simulink model "IntecoVirtualDrl"  (R2020b)
settings: Solver=ode5  StartTime=0.0  StopTime=inf  FixedStep=0.01  RelTol=1e-3  AbsTol=1e-6
undefined symbols (not defined in the file): Standard_Devices, UDP_Protocol
libraries: sldrtlib x3, simulink x1
settings Model: SimulationMode=external  ExtModeTrigDuration=18000  ExtModeTrigLevel=0.400000  Creator=jims  LastModifiedBy=Mark
settings SolverCC: AutoScaleAbsTol=off
settings DataIOCC: ExternalInput=[]  InitialState=[]  MaxDataPoints=5000  SaveFormat=Array  SignalLoggingSaveFormat=ModelDataLogs  SaveOutput=off  SaveTime=off  ReturnWorkspaceOutputs=off
settings OptimizationCC: BooleanDataType=off  ExpressionDepthLimit=2147483647  LifeSpan=inf
settings DebuggingCC: SaveWithParameterizedLinksMsg=none  UnderspecifiedInitializationDetection=Classic  MergeDetectMultiDrivingBlocksExec=none  SignalResolutionControl=TryResolveAllWithWarning  MultiTaskDSMMsg=warning  MultiTaskCondExecSysMsg=none  IntegerOverflowMsg=none  FcnCallInpInsideContextMsg=warning  StateNameClashWarn=warning  SFUnexpectedBacktrackingDiag=warning  SFNoUnconditionalDefaultTransitionDiag=warning  SFExecutionAtInitializationDiag=none  IntegerSaturationMsg=none  ArithmeticOperatorsInVariantConditions=warning
settings HardwareCC: TargetBitPerLong=64  TargetBitPerPointer=64  TargetIntDivRoundTo=Zero  TargetEndianess=LittleEndian  TargetWordSize=64  TargetHWDeviceType=Intel->x86-64
settings ModelReferenceCC: PropagateSignalLabelsOutOfModel=off
settings SFSimCC: SimUseLocalCustomCode=off  CustomCodeUndefinedFunction=UseInterfaceOnly
settings RTWCC: Description=Simulink Desktop Real-Time  SystemTargetFile=sldrt.tlc  TemplateMakefile=sldrt.tmf  RTWUseLocalCustomCode=off  RTWCompilerOptimization=on
settings CodeAppCC: MaxIdLength=95  StateflowObjectComments=on
settings SimulinkDesktopRealTimeCC: TargetPreCompLibLocation=C:\Program Files\MATLAB\R2020b\toolbox\sldrt\lib\win64  TargetLangStandard=C89/C90 (ANSI)  SupportVariableSizeSignals=off
settings ConfigComp: CovMetricSettings=dw  CovSaveCumulativeToWorkspaceVar=on  CovSaveSingleToWorkspaceVar=on  CovExternalEMLEnable=off

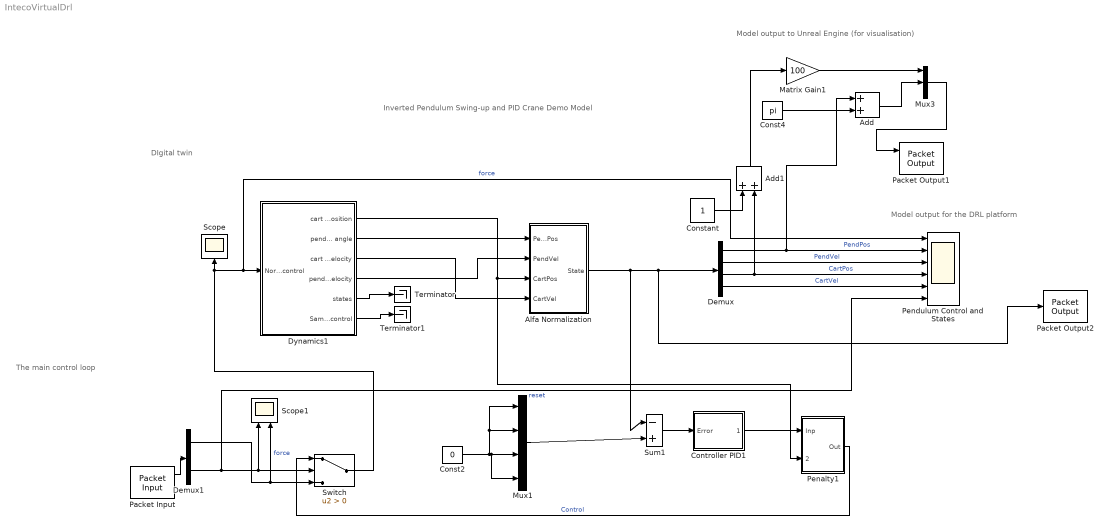
== system IntecoVirtualDrl ==
  note: Model output for the DRL platform
  note: Model output to Unreal Engine (for visualisation)
  note: DIgital twin
  note: The main control loop
  note: Inverted Pendulum
      | Swing-up and PID Crane Demo Model
  Add : Sum
  Add1 : Sum
  Alfa Normalization : Subsystem  mask(Choose mode:){}
  Const2 : Constant  Value=0
  Const4 : Constant  Value=pi
  Constant : Constant
  Controller PID1 : Subsystem  mask{Cart_PID=[ -0.8 0 -0.05 ], Pend_PID=[ -1 0 -0.0 ], Umax=0.5, zone=1.3, Friction=0.05, T0=0.01}
      mask prompts: Cart_PID "Cart PID parameters [Kp, Ki, Kd]:"; Pend_PID "Pendulum PID parameters [Kp, Ki, Kd]:"; Umax "Maximum control value:"; zone "Stabilisation zone [rad]:"; Friction "Friction compensation:"; T0 "Sample time:"
  Demux : Demux
      settings: DisplayOption=none
  Demux1 : Demux  Outputs=2
      settings: DisplayOption=none
  Dynamics1 : Subsystem  mask(Dynamics){x_ini=[0, 3.132388768862475, 0.002930656000000, 0.003140672265117062], m=[0.572066, 0.119648], fr=[0.000276, 1.199442, 0.502926], P4=[0.019631, 0.003861, 9.826466], Up=[6.338787, 0.227417], DZ=[0.099952, 1.495618]}
      mask prompts: x_ini "Initial state vector [x1(0)  x2(0)  x3(0)  x4(0)]"; m "mass of cart (mc)  mass of pendulum (mp)"; fr "friction :  fp  FS  FC"; P4 "Distance (l), Total Inertia moment (J), gravity (g)"; Up "control : magnitude (M)    DZu"; DZ "minimal velocities : cart (DZcv)  pendulum (DZcp)"
      mask help:
      | Pendulum-Cart Dynamics
      |
      | Copyright INTECO 1997
      mask init:
      | DZcv=DZ(1);DZcp=DZ(2);DZu=Up(2);l=P4(1);J=P4(2);g=P4(3);M=Up(1);mc=m(1);mp=m(2);fp=fr(1);FS=fr(2);FC=fr(3);mi=l*(mc+mp);a=l*l+J/(mc+mp);
      mask Display: plot(0,0,100,100,[40,48,48,40,40],[60,60,49,49,60],[37,44],[9,54],[100,8,4,1,0,100,100,0,40,100,100,0,0,40],[44,44,44,44,45,46,45,44,45,45,43,43,46,46],[100,48],[55,55],[0,40],[55,55])
  Matrix Gain1 : Gain  Gain=100  SaturateOnIntegerOverflow=on  OutDataTypeStr=Inherit: Same as input  ParamDataTypeStr=Inherit: Same as input
  Mux1 : Mux
  Mux3 : Mux  Inputs=3
  Packet Input : sldrtlib/Packet Input  SampleTime=0.03  MaxMissedTicks=10  ShowMissedTicks=off  YieldWhenWaiting=off  DrvName=Standard_Devices/UDP_Protocol  DrvAddress=16384  DrvOptions=[0 16384 49 50 55 46 48 46 48 46 49 0 0 0 0 0 0 0 0 0 0 0 0 0 0 0 0 0 0 0 0 0 0 0 0 0 0 0 0 0 0 0 0 0 0 0 0 0 0 0 0 0 0 0 0 0 0 0 0 0 0 0 0 0 0 0 0 0 0 0 0 0 0 0 0 0 0 0 0 0 0 0 0 0 0 0 0 0 0 0 0 0 0 0 0 0 0 0 0 0 0 0 0 0 0 0 0 0 0 0 0 0 0 0 0 0 0 0 0 0 0 0 0 0 0 0 0 0 0 0 0 0 0 0 0 0 0 0 0 0 0 0 0 0 0 0 0 0 0 0 0 0 0 0 0 0 0 0 0 0 0 0 0 0 0 0 0 0 0 0 0 0 0 0 0 0 0 0 0 0 0 0 0 0 0 0 0 0 0 0 0 0 0 0 0 0 0 0 0 0 0 0 0 0 0 0 0 0 0 0 0 0 0 0 0 0 0 0 0 0 0 0 0 0 0 0 0 0 0 0 0 0 0 0 0 0 0 0 0 0 0 0 0 0 0 0 0 0 0 0 0 0 0 0 0 0]  PacketSize=16  DataTypes='2*double'  ShowReady=on  ShowError=off  PacketID=1  ByteOrder=2  ShowTimestamp=off
      settings: AttributesFormatString=UDP Protocol [16384]
  Packet Output1 : sldrtlib/Packet Output  SampleTime=0.03  MaxMissedTicks=25  ShowMissedTicks=on  YieldWhenWaiting=off  DrvName=Standard_Devices/UDP_Protocol  DrvAddress=9999  DrvOptions=[0 8888 49 50 55 46 48 46 48 46 49 0 0 0 0 0 0 0 0 0 0 0 0 0 0 0 0 0 0 0 0 0 0 0 0 0 0 0 0 0 0 0 0 0 0 0 0 0 0 0 0 0 0 0 0 0 0 0 0 0 0 0 0 0 0 0 0 0 0 0 0 0 0 0 0 0 0 0 0 0 0 0 0 0 0 0 0 0 0 0 0 0 0 0 0 0 0 0 0 0 0 0 0 0 0 0 0 0 0 0 0 0 0 0 0 0 0 0 0 0 0 0 0 0 0 0 0 0 0 0 0 0 0 0 0 0 0 0 0 0 0 0 0 0 0 0 0 0 0 0 0 0 0 0 0 0 0 0 0 0 0 0 0 0 0 0 0 0 0 0 0 0 0 0 0 0 0 0 0 0 0 0 0 0 0 0 0 0 0 0 0 0 0 0 0 0 0 0 0 0 0 0 0 0 0 0 0 0 0 0 0 0 0 0 0 0 0 0 0 0 0 0 0 0 0 0 0 0 0 0 0 0 0 0 0 0 0 0 0 0 0 0 0 0 0 0 0 0 0 0 0 0 0 0 0 0]  PacketSize=83  DataTypes={'20*single', '3*uint8'}  ShowReady=off  ShowError=off  PacketID=1  ByteOrder=1  InitialValue=[]  FinalValue=[]
      settings: AttributesFormatString=UDP Protocol [9999]
  Packet Output2 : sldrtlib/Packet Output  SampleTime=0.03  MaxMissedTicks=25  ShowMissedTicks=on  YieldWhenWaiting=off  DrvName=Standard_Devices/UDP_Protocol  DrvAddress=16385  DrvOptions=[0 16385 49 50 55 46 48 46 48 46 49 0 0 0 0 0 0 0 0 0 0 0 0 0 0 0 0 0 0 0 0 0 0 0 0 0 0 0 0 0 0 0 0 0 0 0 0 0 0 0 0 0 0 0 0 0 0 0 0 0 0 0 0 0 0 0 0 0 0 0 0 0 0 0 0 0 0 0 0 0 0 0 0 0 0 0 0 0 0 0 0 0 0 0 0 0 0 0 0 0 0 0 0 0 0 0 0 0 0 0 0 0 0 0 0 0 0 0 0 0 0 0 0 0 0 0 0 0 0 0 0 0 0 0 0 0 0 0 0 0 0 0 0 0 0 0 0 0 0 0 0 0 0 0 0 0 0 0 0 0 0 0 0 0 0 0 0 0 0 0 0 0 0 0 0 0 0 0 0 0 0 0 0 0 0 0 0 0 0 0 0 0 0 0 0 0 0 0 0 0 0 0 0 0 0 0 0 0 0 0 0 0 0 0 0 0 0 0 0 0 0 0 0 0 0 0 0 0 0 0 0 0 0 0 0 0 0 0 0 0 0 0 0 0 0 0 0 0 0 0 0 0 0 0 0 0]  PacketSize=32  DataTypes='4*double'  ShowReady=off  ShowError=off  PacketID=1  ByteOrder=2  InitialValue=[]  FinalValue=[]
      settings: AttributesFormatString=UDP Protocol [16385]
  Penalty1 : Subsystem
  Pendulum Control and States : Scope  NumInputPorts=6
  Scope : Scope
  Scope1 : Scope  NumInputPorts=2
  Sum1 : Sum  Inputs=|-+  InputSameDT=on  SaturateOnIntegerOverflow=on  OutDataTypeStr=Inherit: Same as first input
  Switch : Switch  Criteria=u2 > Threshold
  Terminator : Terminator
  Terminator1 : Terminator
  wires:
  Demux/4 -> Pendulum Control and States/5  "CartVel"
  Demux/3 -> Pendulum Control and States/4, Add1/2  "CartPos"
  Demux/2 -> Pendulum Control and States/3  "PendVel"
  Demux/1 -> Add/1, Pendulum Control and States/2  "PendPos"
  Dynamics1/2(pendulum angle) -> Alfa Normalization/1(PendPos)
  Dynamics1/4(pendulum velocity) -> Alfa Normalization/2(PendVel)
  Dynamics1/1(cart position) -> Penalty1/2(CartPos), Alfa Normalization/3(CartPos)
  Dynamics1/3(cart velocity) -> Alfa Normalization/4(CartVel)
  Dynamics1/5(states) -> Terminator/1
  Dynamics1/6(Sampled control) -> Terminator1/1
  Mux3/1 -> Packet Output1/1
  Matrix Gain1/1 -> Mux3/1
  Const4/1 -> Add/2
  Add/1 -> Mux3/2
  Sum1/1 -> Controller PID1/1(Error)
  Packet Input/1 -> Demux1/1
  Demux1/2 -> Pendulum Control and States/6, Scope1/1, Switch/2  "reset"
  Demux1/1 -> Switch/3, Scope1/2  "force"
  Switch/1 -> Dynamics1/1(Normalized control), Pendulum Control and States/1, Scope/1  "force"
  Constant/1 -> Add1/1
  Add1/1 -> Matrix Gain1/1
  Const2/1 -> Mux1/1, Mux1/2, Mux1/4, Mux1/3
  Mux1/1 -> Sum1/2
  Controller PID1/1(Control) -> Penalty1/1(Inp)
  Alfa Normalization/1(State) -> Sum1/1, Packet Output2/1, Demux/1
  Penalty1/1(Out) -> Switch/1  "Control"

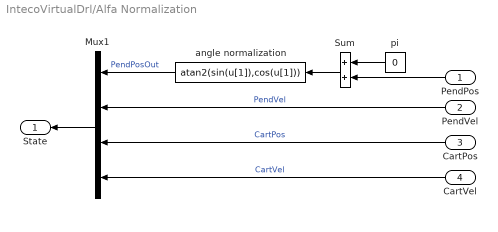
== system IntecoVirtualDrl/Alfa Normalization ==
  PendPos : Inport
  PendVel : Inport  Port=2
  CartPos : Inport  Port=3
  CartVel : Inport  Port=4
  Mux1 : Mux
  Sum : Sum  InputSameDT=on  SaturateOnIntegerOverflow=on  OutDataTypeStr=Inherit: Same as first input
  angle normalization : Fcn  Expr=atan2(sin(u[1]),cos(u[1]))
  pi : Constant  Value=0
  State : Outport  InitialOutput=0  VectorParamsAs1DForOutWhenUnconnected=off
  wires:
  pi/1 -> Sum/1
  Sum/1 -> angle normalization/1
  Mux1/1 -> State/1
  CartPos/1 -> Mux1/3  "CartPos"
  CartVel/1 -> Mux1/4  "CartVel"
  PendVel/1 -> Mux1/2  "PendVel"
  PendPos/1 -> Sum/2
  angle normalization/1 -> Mux1/1  "PendPosOut"

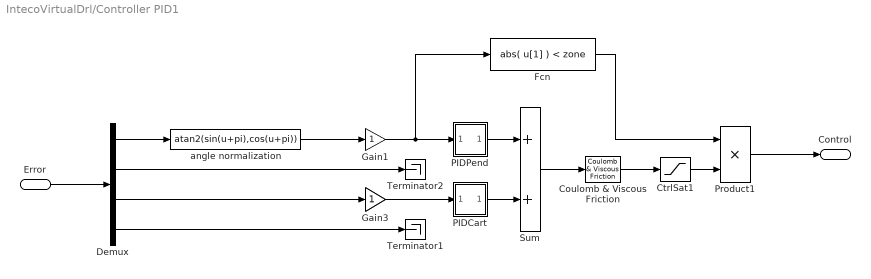
== system IntecoVirtualDrl/Controller PID1 ==
  Error : Inport
  Coulomb & Viscous Friction : simulink/Discontinuities/Coulomb & Viscous Friction  offset=Friction  gain=1
  CtrlSat1 : Saturate  UpperLimit=Umax  LowerLimit=-Umax
  Demux : Demux
      settings: DisplayOption=none
  Fcn : Fcn  Expr=abs( u[1] ) < zone
  Gain1 : Gain  SaturateOnIntegerOverflow=on  OutDataTypeStr=Inherit: Same as input  ParamDataTypeStr=Inherit: Same as input
  Gain3 : Gain  SaturateOnIntegerOverflow=on  OutDataTypeStr=Inherit: Same as input  ParamDataTypeStr=Inherit: Same as input
  PIDCart : Subsystem  mask(PID(2) Controller){P=Cart_PID(1), I=Cart_PID(2), D=Cart_PID(3), T0=T0}
      mask prompts: P "Proportional:"; I "Integral:"; D "Derivative:"; T0 "Sample Time:"
      mask help:
      | Enter Proportional(P), Integral(I), and Derivative(D) and divisor (N) terms.
      | P+I/s+Ds/(1/Ns+1)
      mask Help: This block implements a PID controller where parameters are entered for the Proportional, Integral and Derivative and divisor terms. Unmask this block to see how it works. The derivative term is implemented using an s/(s/N +1)  transfer function block. Making N large can create a "stiff" system.
      mask Display: disp('PID')
  PIDPend : Subsystem  mask(PID(2) Controller){P=Pend_PID(1), I=Pend_PID(2), D=Pend_PID(3), T0=T0}
      mask prompts: P "Proportional:"; I "Integral:"; D "Derivative:"; T0 "Sample Time:"
      mask help:
      | Enter Proportional(P), Integral(I), and Derivative(D) and divisor (N) terms.
      | P+I/s+Ds/(1/Ns+1)
      mask Help: This block implements a PID controller where parameters are entered for the Proportional, Integral and Derivative and divisor terms. Unmask this block to see how it works. The derivative term is implemented using an s/(s/N +1)  transfer function block. Making N large can create a "stiff" system.
      mask Display: disp('PID')
  Product1 : Product  InputSameDT=on  RndMeth=Zero  SaturateOnIntegerOverflow=on  OutDataTypeStr=Inherit: Same as first input
  Sum : Sum  InputSameDT=on  SaturateOnIntegerOverflow=on  OutDataTypeStr=Inherit: Same as first input
  Terminator1 : Terminator
  Terminator2 : Terminator
  angle normalization : Fcn  Expr=atan2(sin(u+pi),cos(u+pi))
  Control : Outport  InitialOutput=0  VectorParamsAs1DForOutWhenUnconnected=off
  wires:
  angle normalization/1 -> Gain1/1
  PIDCart/1(Out_1) -> Sum/2
  Gain3/1 -> PIDCart/1(In_1)
  Product1/1 -> Control/1
  Fcn/1 -> Product1/1
  CtrlSat1/1 -> Product1/2
  Coulomb & Viscous Friction/1 -> CtrlSat1/1
  Sum/1 -> Coulomb & Viscous Friction/1
  PIDPend/1(Out_1) -> Sum/1
  Gain1/1 -> PIDPend/1(In_1), Fcn/1
  Demux/1 -> angle normalization/1
  Error/1 -> Demux/1
  Demux/2 -> Terminator2/1
  Demux/3 -> Gain3/1
  Demux/4 -> Terminator1/1

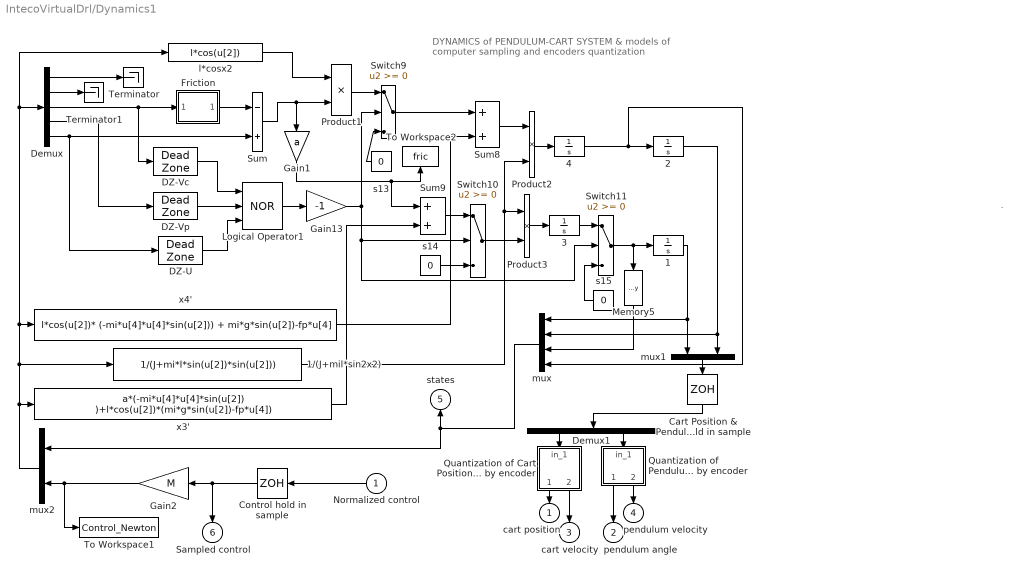
== system IntecoVirtualDrl/Dynamics1 ==
  note: DYNAMICS of
      | PENDULUM-CART SYSTEM
      | & models of
      | computer sampling and encoders quantization
  note: .
  Normalized control : Inport
  " Quantization of Pendulum Angle introduced by encoder" : Subsystem
  1 : Integrator  InitialCondition=x_ini(1)
  1/(J+mil*sin2x2) : Fcn  Expr=1/(J+mi*l*sin(u[2])*sin(u[2]))
  2 : Integrator  InitialCondition=x_ini(2)
  3 : Integrator  InitialCondition=x_ini(3)
  4 : Integrator  InitialCondition=x_ini(4)
  Cart Position & Pendulum Angle hold in sample : ZeroOrderHold  SampleTime=0.01
  Control hold in sample : ZeroOrderHold  SampleTime=0.01
  DZ-U : DeadZone  LowerValue=-DZu  UpperValue=DZu  SaturateOnIntegerOverflow=on
  DZ-Vc : DeadZone  LowerValue=-DZcv  UpperValue=DZcv  SaturateOnIntegerOverflow=on
  DZ-Vp : DeadZone  LowerValue=-DZcp  UpperValue=DZcp  SaturateOnIntegerOverflow=on
  Demux : Demux  Outputs=5
      settings: DisplayOption=none
  Demux1 : Demux  Outputs=2
      settings: DisplayOption=none
  Friction : Subsystem  mask(Coulombic and Viscous Friction){FS=FS, FC=FC}
      mask prompts: FS "Static friction"; FC "Coulomb friction"
      mask help:
      | A discontinuity offset at zero models coulomb friction.  Linear gain models viscous friction.
      | y = sign(x) * (Umax * abs(x) + friction)
      mask Help:
      | This block has a discontinuity
      | at zero and a linear gain afterward.
      | y= sign(x)*(Umax*abs(x)+friction)
  Gain1 : Gain  Gain=a  SaturateOnIntegerOverflow=on  OutDataTypeStr=Inherit: Same as input  ParamDataTypeStr=Inherit: Same as input
  Gain13 : Gain  Gain=-1  SaturateOnIntegerOverflow=on  OutDataTypeStr=Inherit: Same as input  ParamDataTypeStr=Inherit: Same as input
  Gain2 : Gain  Gain=M  SaturateOnIntegerOverflow=on  OutDataTypeStr=Inherit: Same as input  ParamDataTypeStr=Inherit: Same as input
  Logical Operator1 : Logic  Operator=NOR  Inputs=3
  Memory5 : Memory
  Product1 : Product  InputSameDT=on  RndMeth=Zero  SaturateOnIntegerOverflow=on  OutDataTypeStr=Inherit: Same as first input
  Product2 : Product  InputSameDT=on  RndMeth=Zero  SaturateOnIntegerOverflow=on  OutDataTypeStr=Inherit: Same as first input
  Product3 : Product  InputSameDT=on  RndMeth=Zero  SaturateOnIntegerOverflow=on  OutDataTypeStr=Inherit: Same as first input
  "Quantization of Cart Position introduced by encoder " : Subsystem
  Sum : Sum  Inputs=-+  InputSameDT=on  SaturateOnIntegerOverflow=on  OutDataTypeStr=Inherit: Same as first input
  Sum8 : Sum  InputSameDT=on  SaturateOnIntegerOverflow=on  OutDataTypeStr=Inherit: Same as first input
  Sum9 : Sum  InputSameDT=on  SaturateOnIntegerOverflow=on  OutDataTypeStr=Inherit: Same as first input
  Switch10 : Switch  SaturateOnIntegerOverflow=on  InputSameDT=on
  Switch11 : Switch  SaturateOnIntegerOverflow=on  InputSameDT=on
  Switch9 : Switch  SaturateOnIntegerOverflow=on  InputSameDT=on
  Terminator : Terminator
  Terminator1 : Terminator
  To Workspace1 : ToWorkspace  VariableName=Control_Newton
      settings: MaxDataPoints=100000
  To Workspace2 : ToWorkspace  VariableName=fric
      settings: MaxDataPoints=100000
  l*cosx2 : Fcn  Expr=l*cos(u[2])
  mux : Mux
  mux1 : Mux  Inputs=2
  mux2 : Mux  Inputs=[4 1]
  s13 : Constant  Value=0
  s14 : Constant  Value=0
  s15 : Constant  Value=0
  x3' : Fcn  Expr=a*(-mi*u[4]*u[4]*sin(u[2]) )+l*cos(u[2])*(mi*g*sin(u[2])-fp*u[4])
  x4' : Fcn  Expr=l*cos(u[2])* (-mi*u[4]*u[4]*sin(u[2])) + mi*g*sin(u[2])-fp*u[4]
  cart position : Outport  InitialOutput=0
  pendulum angle : Outport  Port=2  InitialOutput=0
  cart velocity : Outport  Port=3  InitialOutput=0
  pendulum velocity : Outport  Port=4  InitialOutput=0
  states : Outport  Port=5  InitialOutput=0
  Sampled control : Outport  Port=6  InitialOutput=0
  wires:
  Demux1/1 -> "Quantization of Cart Position introduced by encoder "/1(in_1)
  mux/1 -> mux2/1, states/1
  "Quantization of Cart Position introduced by encoder "/1(out_1) -> cart position/1
  "Quantization of Cart Position introduced by encoder "/2(out_2) -> cart velocity/1
  " Quantization of Pendulum Angle introduced by encoder"/1(out_1) -> pendulum angle/1
  " Quantization of Pendulum Angle introduced by encoder"/2(out_2) -> pendulum velocity/1
  Demux1/2 -> " Quantization of Pendulum Angle introduced by encoder"/1(in_1)
  Control hold in sample/1 -> Sampled control/1, Gain2/1
  Normalized control/1 -> Control hold in sample/1
  Cart Position & Pendulum Angle hold in sample/1 -> Demux1/1
  mux1/1 -> Cart Position & Pendulum Angle hold in sample/1
  2/1 -> mux1/2, mux/2
  4/1 -> mux/4, 2/1
  Switch11/1 -> Memory5/1, 1/1
  Demux/2 -> Terminator1/1
  Demux/5 -> DZ-U/1, Sum/2
  Demux/1 -> Terminator/1
  Demux/4 -> DZ-Vp/1
  Demux/3 -> DZ-Vc/1, Friction/1(In1)
  DZ-U/1 -> Logical Operator1/3
  Logical Operator1/1 -> Gain13/1
  DZ-Vp/1 -> Logical Operator1/2
  DZ-Vc/1 -> Logical Operator1/1
  l*cosx2/1 -> Product1/1
  s13/1 -> Switch9/3
  Switch9/1 -> Sum8/1
  s14/1 -> Switch10/3
  Product1/1 -> Switch9/1
  x4'/1 -> Sum8/2
  Sum8/1 -> Product2/1
  Product2/1 -> 4/1
  Sum9/1 -> Switch10/1
  3/1 -> Switch11/1
  s15/1 -> Switch11/3
  Gain13/1 -> Switch9/2, Switch11/2, Switch10/2
  Switch10/1 -> Product3/2
  Sum/1 -> Product1/2, Gain1/1
  mux2/1 -> x3'/1, Demux/1, l*cosx2/1, x4'/1, 1/(J+mil*sin2x2)/1
  x3'/1 -> Sum9/2
  1/(J+mil*sin2x2)/1 -> Product2/2, Product3/1
  Gain1/1 -> Sum9/1, To Workspace2/1
  Gain2/1 -> To Workspace1/1, mux2/2
  Friction/1(Out1) -> Sum/1
  Product3/1 -> 3/1
  1/1 -> mux1/1, mux/1
  Memory5/1 -> mux/3

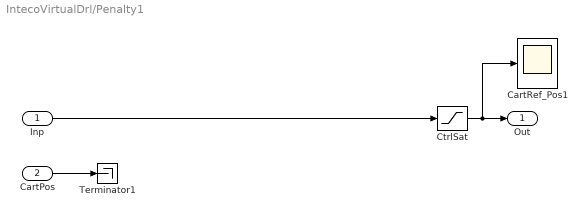
== system IntecoVirtualDrl/Penalty1 ==
  Inp : Inport
  CartPos : Inport  Port=2
  CartRef_Pos1 : Scope
  CtrlSat : Saturate
  Terminator1 : Terminator
  Out : Outport  VectorParamsAs1DForOutWhenUnconnected=off
  wires:
  CtrlSat/1 -> Out/1, CartRef_Pos1/1
  Inp/1 -> CtrlSat/1
  CartPos/1 -> Terminator1/1

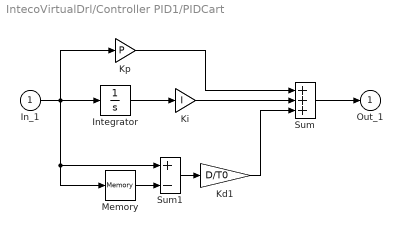
== system IntecoVirtualDrl/Controller PID1/PIDCart ==
  In_1 : Inport
  Integrator : Integrator  LimitOutput=on  UpperSaturationLimit=1  LowerSaturationLimit=-1
  Kd1 : Gain  Gain=D/T0  SaturateOnIntegerOverflow=on  OutDataTypeStr=Inherit: Same as input  ParamDataTypeStr=Inherit: Same as input
  Ki : Gain  Gain=I  SaturateOnIntegerOverflow=on  OutDataTypeStr=Inherit: Same as input  ParamDataTypeStr=Inherit: Same as input
  Kp : Gain  Gain=P  SaturateOnIntegerOverflow=on  OutDataTypeStr=Inherit: Same as input  ParamDataTypeStr=Inherit: Same as input
  Memory : Memory
  Sum : Sum  Inputs=+++  InputSameDT=on  SaturateOnIntegerOverflow=on  OutDataTypeStr=Inherit: Same as first input
  Sum1 : Sum  Inputs=+-  InputSameDT=on  SaturateOnIntegerOverflow=on  OutDataTypeStr=Inherit: Same as first input
  Out_1 : Outport  InitialOutput=0  VectorParamsAs1DForOutWhenUnconnected=off
  wires:
  Kd1/1 -> Sum/3
  Sum1/1 -> Kd1/1
  Memory/1 -> Sum1/2
  Kp/1 -> Sum/1
  Sum/1 -> Out_1/1
  In_1/1 -> Sum1/1, Memory/1, Kp/1, Integrator/1
  Integrator/1 -> Ki/1
  Ki/1 -> Sum/2

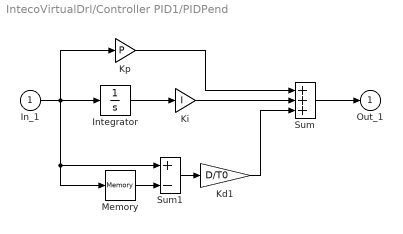
== system IntecoVirtualDrl/Controller PID1/PIDPend ==
  In_1 : Inport
  Integrator : Integrator  LimitOutput=on  UpperSaturationLimit=1  LowerSaturationLimit=-1
  Kd1 : Gain  Gain=D/T0  SaturateOnIntegerOverflow=on  OutDataTypeStr=Inherit: Same as input  ParamDataTypeStr=Inherit: Same as input
  Ki : Gain  Gain=I  SaturateOnIntegerOverflow=on  OutDataTypeStr=Inherit: Same as input  ParamDataTypeStr=Inherit: Same as input
  Kp : Gain  Gain=P  SaturateOnIntegerOverflow=on  OutDataTypeStr=Inherit: Same as input  ParamDataTypeStr=Inherit: Same as input
  Memory : Memory
  Sum : Sum  Inputs=+++  InputSameDT=on  SaturateOnIntegerOverflow=on  OutDataTypeStr=Inherit: Same as first input
  Sum1 : Sum  Inputs=+-  InputSameDT=on  SaturateOnIntegerOverflow=on  OutDataTypeStr=Inherit: Same as first input
  Out_1 : Outport  InitialOutput=0  VectorParamsAs1DForOutWhenUnconnected=off
  wires:
  Ki/1 -> Sum/2
  Integrator/1 -> Ki/1
  In_1/1 -> Integrator/1, Kp/1, Memory/1, Sum1/1
  Sum/1 -> Out_1/1
  Kp/1 -> Sum/1
  Memory/1 -> Sum1/2
  Sum1/1 -> Kd1/1
  Kd1/1 -> Sum/3

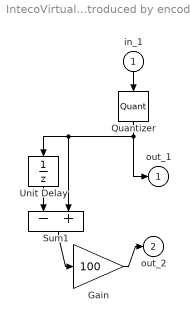
== system IntecoVirtualDrl/Dynamics1/ Quantization of Pendulum Angle introduced by encoder ==
  in_1 : Inport
  Gain : Gain  Gain=100  SaturateOnIntegerOverflow=on  OutDataTypeStr=Inherit: Same as input  ParamDataTypeStr=Inherit: Same as input
  Quantizer : Quantizer  QuantizationInterval=0.001534
  Sum1 : Sum  Inputs=-+  InputSameDT=on  SaturateOnIntegerOverflow=on  OutDataTypeStr=Inherit: Same as first input
  Unit Delay : UnitDelay  InitialCondition=x_ini(2)  SampleTime=0.01  HasFrameUpgradeWarning=on
  out_1 : Outport  InitialOutput=0
  out_2 : Outport  Port=2  InitialOutput=0
  wires:
  in_1/1 -> Quantizer/1
  Quantizer/1 -> Sum1/2, Unit Delay/1, out_1/1
  Sum1/1 -> Gain/1
  Gain/1 -> out_2/1
  Unit Delay/1 -> Sum1/1

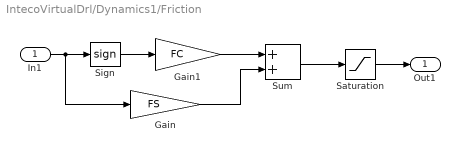
== system IntecoVirtualDrl/Dynamics1/Friction ==
  In1 : Inport
  Gain : Gain  Gain=FS  SaturateOnIntegerOverflow=on  OutDataTypeStr=Inherit: Same as input  ParamDataTypeStr=Inherit: Same as input
  Gain1 : Gain  Gain=FC  SaturateOnIntegerOverflow=on  OutDataTypeStr=Inherit: Same as input  ParamDataTypeStr=Inherit: Same as input
  Saturation : Saturate  UpperLimit=1  LowerLimit=-1
  Sign : Signum
  Sum : Sum  InputSameDT=on  SaturateOnIntegerOverflow=on  OutDataTypeStr=Inherit: Same as first input
  Out1 : Outport  InitialOutput=0
  wires:
  Saturation/1 -> Out1/1
  Sum/1 -> Saturation/1
  Sign/1 -> Gain1/1
  In1/1 -> Gain/1, Sign/1
  Gain1/1 -> Sum/1
  Gain/1 -> Sum/2

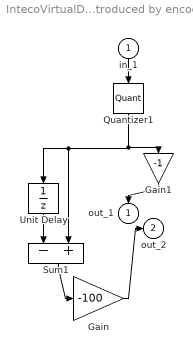
== system IntecoVirtualDrl/Dynamics1/Quantization of Cart Position introduced by encoder  ==
  in_1 : Inport
  Gain : Gain  Gain=-100  SaturateOnIntegerOverflow=on  OutDataTypeStr=Inherit: Same as input  ParamDataTypeStr=Inherit: Same as input
  Gain1 : Gain  Gain=-1
  Quantizer1 : Quantizer  QuantizationInterval=5.7053e-005
  Sum1 : Sum  Inputs=-+  InputSameDT=on  SaturateOnIntegerOverflow=on  OutDataTypeStr=Inherit: Same as first input
  Unit Delay : UnitDelay  InitialCondition=x_ini(1)  SampleTime=0.01  HasFrameUpgradeWarning=on
  out_1 : Outport  InitialOutput=0
  out_2 : Outport  Port=2  InitialOutput=0
  wires:
  Quantizer1/1 -> Gain1/1, Sum1/2, Unit Delay/1
  Unit Delay/1 -> Sum1/1
  Gain/1 -> out_2/1
  in_1/1 -> Quantizer1/1
  Sum1/1 -> Gain/1
  Gain1/1 -> out_1/1
